simulink model "VU_NXTWay_Simple"  (Simulink 7.5)
settings: Solver=FixedStepDiscrete  SolverMode=SingleTasking  StartTime=0.0  StopTime=inf  FixedStep=0.004  RelTol=1e-3
PreLoadFcn:
  | param_plant, param_controller
values from neighbouring files (symbols this model uses):
  a_b = 0.8    [param_controller.m]
  a_d = 0.8    [param_controller.m]
  a_gc = 0.8    [param_controller.m]
  a_gd = 0.999    [param_controller.m]
  a_r = 0.996    [param_controller.m]
  gp_max = 100    [param_controller.m]
  k_f = KK(1, 1:4)    [param_controller.m]
  k_i = KK(1, 5)    [param_controller.m]
  k_phidot = 25    [param_controller.m]
  k_sync = 0.35    [param_controller.m]
  k_thetadot = 0.3 / R    [param_controller.m]
  pwm_gain = 1    [param_controller.m]
  sound_freq = 440    [param_controller.m]
  time_start = 1000    [param_controller.m]
  ts1 = 0.004    [param_controller.m]
libraries: lego_nxt_lib x8, simulink x3
settings Model: Creator=jpeytonj  LastModifiedBy=jpeytonj
settings DebuggingCC: SingleTaskRateTransMsg=warning  Int32ToFloatConvMsg=none  ParameterPrecisionLossMsg=none
settings RTWCC: SystemTargetFile=lrt.tlc  GenCodeOnly=on  TemplateMakefile=lrt_ecrobot.tmf  Description=Lego NXT Real-Time Target  ProcessScript=lrt_make_rtw_hook
settings STFCustomTargetCC: ModelReferenceCompliant=off  GeneratePreprocessorConditionals=Disable all  MatFileLogging=on  SystemTargetFile=lrt.tlc
settings GRTTargetCC: ModelReferenceCompliant=off  ParMdlRefBuildCompliant=off  CompOptLevelCompliant=off  ExtModeMexFile=ext_serial_win32_comm
settings CustomProperty: DataType=RTWOptions_EnumType_C__LegoMindstorms_VU-LRT_lrt_1codeGenType  Value=Integer-only
settings EnumStrPairs: String=Integer-only

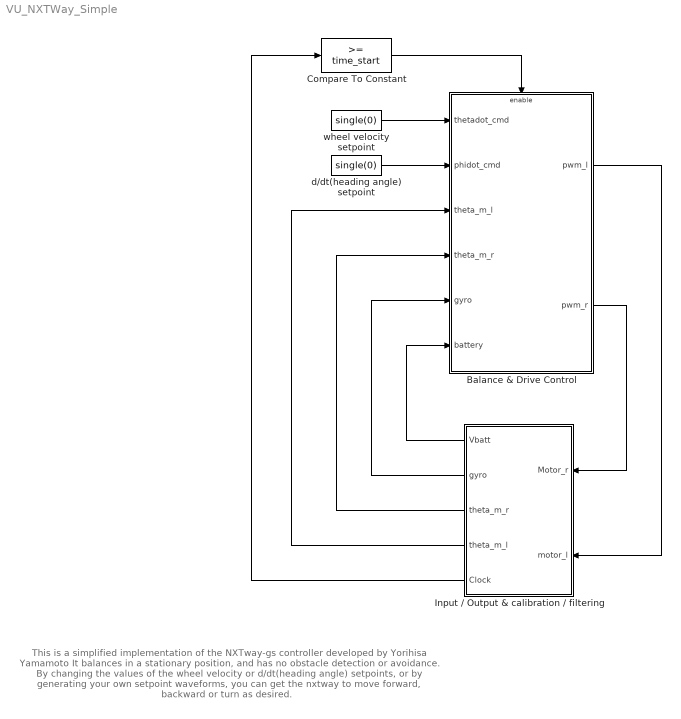
== system VU_NXTWay_Simple ==
  note: This is a simplified implementation of the NXTway-gs controller developed by Yorihisa Yamamoto
      | It balances in a stationary position, and has no obstacle detection or avoidance.
      |
      | By changing the values of the wheel velocity or d/dt(heading angle) setpoints, or by generating
      | your own setpoint waveforms, you can get the nxtway to move forward, backward or turn as desired.
  Balance & Drive Control : Subsystem
  Compare To Constant : simulink/Logic and Bit Operations/Compare To Constant  SystemSampleTime=-1  relop=>=  const=time_start  LogicOutDataTypeMode=boolean
  Input / Output & calibration / filtering : Subsystem
  d/dt(heading angle) setpoint : Constant  Value=single(0)  OutDataType=fixdt(1, 16)  OutScaling=2^0  SampleTime=ts1
  wheel velocity setpoint : Constant  Value=single(0)  OutDataType=fixdt(1, 16)  OutScaling=2^0  SampleTime=ts1
  wires:
  Input / Output & calibration / filtering/1(Vbatt) -> Balance & Drive Control/6(battery)
  Balance & Drive Control/2(pwm_r) -> Input / Output & calibration / filtering/1(Motor_r)
  Balance & Drive Control/1(pwm_l) -> Input / Output & calibration / filtering/2(motor_l)
  Compare To Constant/1 -> Balance & Drive Control/Enable
  Input / Output & calibration / filtering/5(Clock) -> Compare To Constant/1
  Input / Output & calibration / filtering/2(gyro) -> Balance & Drive Control/5(gyro)
  Input / Output & calibration / filtering/3(theta_m_r) -> Balance & Drive Control/4(theta_m_r)
  Input / Output & calibration / filtering/4(theta_m_l) -> Balance & Drive Control/3(theta_m_l)
  d/dt(heading angle) setpoint/1 -> Balance & Drive Control/2(phidot_cmd)
  wheel velocity setpoint/1 -> Balance & Drive Control/1(thetadot_cmd)

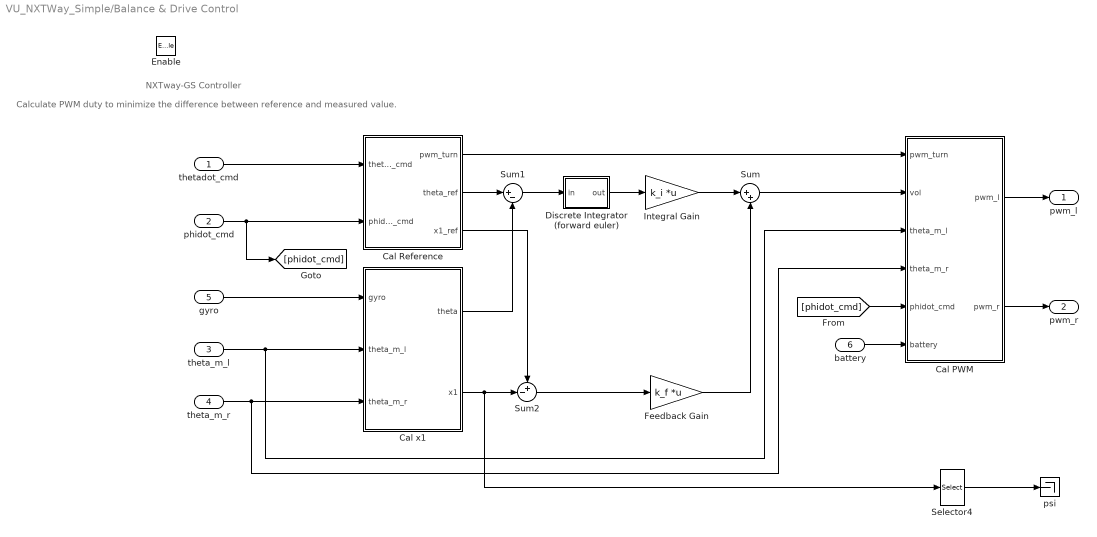
== system VU_NXTWay_Simple/Balance & Drive Control ==
  note: Calculate PWM duty to minimize the difference between reference and measured value.
  note: NXTway-GS Controller
  thetadot_cmd : Inport
  phidot_cmd : Inport  Port=2
  theta_m_l : Inport  Port=3
  theta_m_r : Inport  Port=4
  gyro : Inport  Port=5
  battery : Inport  Port=6
  Enable : EnablePort
  Cal PWM : Subsystem
  Cal Reference : Subsystem
  Cal x1 : Subsystem
  Discrete Integrator (forward euler) : Subsystem
  Feedback Gain : Gain  Gain=k_f  Multiplication=Matrix(K*u)  ParameterDataType=sfix(16)  ParameterScaling=2^0  OutDataType=sfix(16)  OutScaling=2^0  OutDataTypeStr=Inherit: Same as input  ParamDataTypeStr=Inherit: Same as input
  Integral Gain : Gain  Gain=k_i  Multiplication=Matrix(K*u)  ParameterDataType=sfix(16)  ParameterScaling=2^0  OutDataType=sfix(16)  OutScaling=2^0  OutDataTypeStr=Inherit: Same as input  ParamDataTypeStr=Inherit: Same as input
  Selector4 : Selector  InputPortWidth=4  IndexOptions=Index vector (dialog)  Indices=2  OutputSizes=1
  Sum : Sum  Inputs=|++  OutDataType=sfix(16)  OutScaling=2^0  OutDataTypeStr=Inherit: Same as first input
  Sum1 : Sum  Inputs=|+-  OutDataType=sfix(16)  OutScaling=2^0  OutDataTypeStr=Inherit: Same as first input
  Sum2 : Sum  Inputs=+-|  OutDataType=sfix(16)  OutScaling=2^0  OutDataTypeStr=Inherit: Same as first input
  psi : Terminator
  pwm_l : Outport
  pwm_r : Outport  Port=2
  wires:
  [phidot_cmd] -> Cal PWM/5(phidot_cmd)
  Selector4/1 -> psi/1
  Cal Reference/3(x1_ref) -> Sum2/1
  Sum2/1 -> Feedback Gain/1
  Cal x1/2(x1) -> Selector4/1, Sum2/2
  Integral Gain/1 -> Sum/1
  Discrete Integrator (forward euler)/1(out) -> Integral Gain/1
  Sum1/1 -> Discrete Integrator (forward euler)/1(in)
  Cal x1/1(theta) -> Sum1/2
  Cal Reference/2(theta_ref) -> Sum1/1
  Feedback Gain/1 -> Sum/2
  theta_m_r/1 -> Cal PWM/4(theta_m_r), Cal x1/3(theta_m_r)
  battery/1 -> Cal PWM/6(battery)
  Sum/1 -> Cal PWM/2(vol)
  phidot_cmd/1 -> [phidot_cmd], Cal Reference/2(phidot_cmd)
  thetadot_cmd/1 -> Cal Reference/1(thetadot_cmd)
  Cal Reference/1(pwm_turn) -> Cal PWM/1(pwm_turn)
  Cal PWM/1(pwm_l) -> pwm_l/1
  Cal PWM/2(pwm_r) -> pwm_r/1
  theta_m_l/1 -> Cal PWM/3(theta_m_l), Cal x1/2(theta_m_l)
  gyro/1 -> Cal x1/1(gyro)

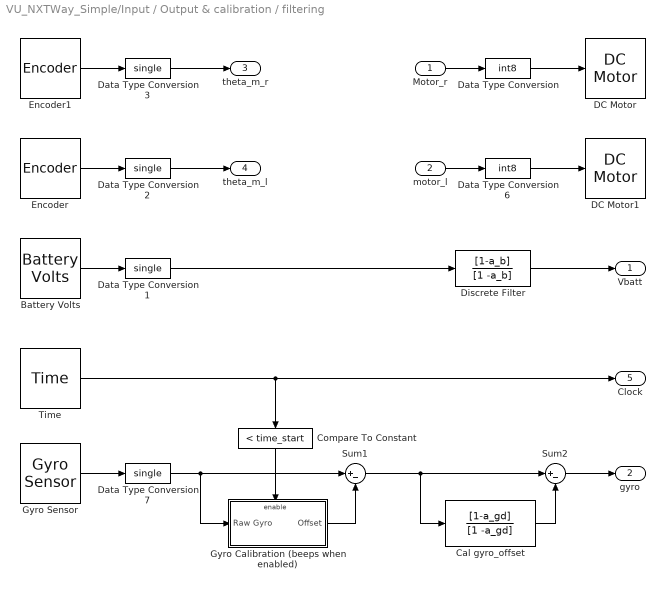
== system VU_NXTWay_Simple/Input / Output & calibration / filtering ==
  Motor_r : Inport
  motor_l : Inport  Port=2
  Battery Volts : lego_nxt_lib/Battery Volts  st=ts3
  Cal gyro_offset : DiscreteFilter  Numerator=[1-a_gd]  Denominator=[1 -a_gd]
  Compare To Constant : simulink/Logic and Bit Operations/Compare To Constant  SystemSampleTime=-1  relop=<  const=time_start  LogicOutDataTypeMode=boolean
  DC Motor : lego_nxt_lib/DC Motor  port=Port C  brake=Brake
  DC Motor1 : lego_nxt_lib/DC Motor  port=Port B  brake=Brake
  Data Type Conversion : DataTypeConversion  OutDataTypeMode=int8  OutDataType=sfix(16)  OutScaling=2^0  OutDataTypeStr=int8  RndMeth=Simplest
      settings: AttributesFormatString=Round = %<RndMeth>
  Data Type Conversion{1..3,7} (4 alike) : DataTypeConversion  OutDataTypeMode=single  OutDataType=sfix(16)  OutScaling=2^0  OutDataTypeStr=single  RndMeth=Simplest
      settings: AttributesFormatString=Round = %<RndMeth>
  Data Type Conversion6 : DataTypeConversion  OutDataTypeMode=int8  OutDataType=sfix(16)  OutScaling=2^0  OutDataTypeStr=int8  RndMeth=Simplest
      settings: AttributesFormatString=Round = %<RndMeth>
  Discrete Filter : DiscreteFilter  Numerator=[1-a_b]  Denominator=[1 -a_b]
  Encoder : lego_nxt_lib/Encoder  port=Port B  st=ts1
  Encoder1 : lego_nxt_lib/Encoder  port=Port C  st=ts1
  Gyro Calibration (beeps when enabled) : Subsystem  TreatAsAtomicUnit=on
  Gyro Sensor : lego_nxt_lib/Gyro Sensor  port=Port 3  st=ts1
  Sum1 : Sum  Inputs=|+-  OutDataType=sfix(16)  OutScaling=2^0  OutDataTypeStr=Inherit: Same as first input
  Sum2 : Sum  Inputs=|+-  OutDataType=sfix(16)  OutScaling=2^0  OutDataTypeStr=Inherit: Same as first input
  Time : lego_nxt_lib/Time  st=ts1
  Vbatt : Outport
  gyro : Outport  Port=2
  theta_m_r : Outport  Port=3
  theta_m_l : Outport  Port=4
  Clock : Outport  Port=5
  wires:
  Gyro Sensor/1 -> Data Type Conversion7/1
  Encoder/1 -> Data Type Conversion2/1
  Encoder1/1 -> Data Type Conversion3/1
  Battery Volts/1 -> Data Type Conversion1/1
  motor_l/1 -> Data Type Conversion6/1
  Motor_r/1 -> Data Type Conversion/1
  Time/1 -> Clock/1, Compare To Constant/1
  Discrete Filter/1 -> Vbatt/1
  Data Type Conversion1/1 -> Discrete Filter/1
  Sum2/1 -> gyro/1
  Data Type Conversion7/1 -> Gyro Calibration (beeps when enabled)/1(Raw Gyro), Sum1/1
  Sum1/1 -> Cal gyro_offset/1, Sum2/1
  Compare To Constant/1 -> Gyro Calibration (beeps when enabled)/Enable
  Cal gyro_offset/1 -> Sum2/2
  Gyro Calibration (beeps when enabled)/1(Offset) -> Sum1/2
  Data Type Conversion2/1 -> theta_m_l/1
  Data Type Conversion3/1 -> theta_m_r/1
  Data Type Conversion/1 -> DC Motor/1
  Data Type Conversion6/1 -> DC Motor1/1

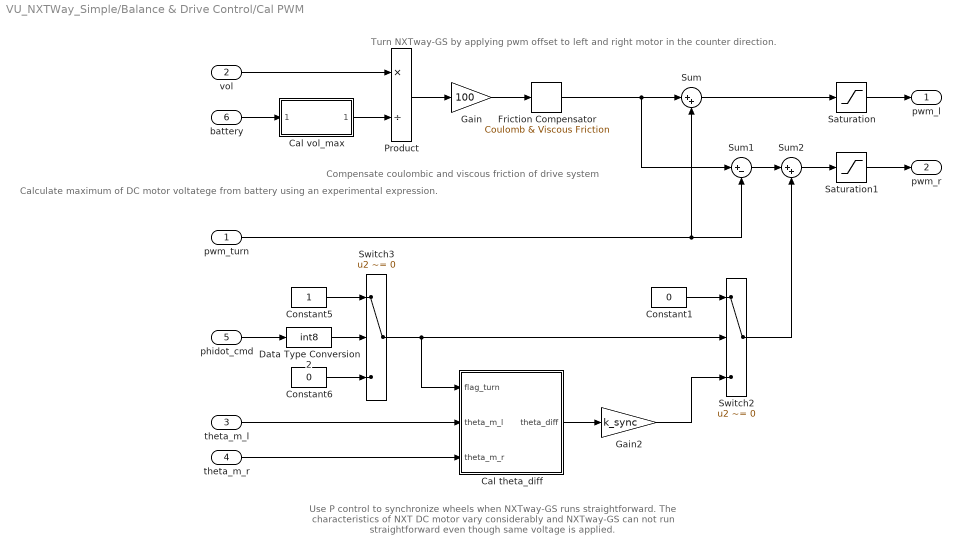
== system VU_NXTWay_Simple/Balance & Drive Control/Cal PWM ==
  note: Compensate coulombic and
      | viscous friction of drive system
  note: Turn NXTway-GS by applying pwm offset
      | to left and right motor in the counter direction.
  note: Use P control to synchronize wheels when NXTway-GS runs straightforward.
      | The characteristics of NXT DC motor vary considerably and NXTway-GS can not
      | run straightforward even though same voltage is applied.
  note: Calculate maximum of DC motor
      | voltatege from battery using an
      | experimental expression.
  pwm_turn : Inport
  vol : Inport  Port=2  OutDataType=sfix(16)  OutScaling=2^0
  theta_m_l : Inport  Port=3  OutDataType=sfix(16)  OutScaling=2^0
  theta_m_r : Inport  Port=4  OutDataType=sfix(16)  OutScaling=2^0
  phidot_cmd : Inport  Port=5
  battery : Inport  Port=6  OutDataType=sfix(16)  OutScaling=2^0
  Cal theta_diff : Subsystem
  Cal vol_max : Subsystem
  Constant1 : Constant  Value=0  OutDataTypeMode=single  OutDataType=sfix(16)  OutScaling=2^0  OutDataTypeStr=single  SampleTime=ts1
      settings: AttributesFormatString=DataType = %<OutDataTypeStr>
  Constant5 : Constant  OutDataTypeMode=boolean  OutDataType=sfix(16)  OutScaling=2^0  OutDataTypeStr=boolean  SampleTime=ts1
      settings: AttributesFormatString=DataType = %<OutDataTypeStr>
  Constant6 : Constant  Value=0  OutDataTypeMode=boolean  OutDataType=sfix(16)  OutScaling=2^0  OutDataTypeStr=boolean  SampleTime=ts1
      settings: AttributesFormatString=DataType = %<OutDataTypeStr>
  Data Type Conversion2 : DataTypeConversion  OutDataTypeMode=int8  OutDataType=sfix(16)  OutScaling=2^0  OutDataTypeStr=int8  RndMeth=Simplest
      settings: AttributesFormatString=Round = %<RndMeth>
  Friction Compensator : simulink/Discontinuities/Coulomb & Viscous Friction  SystemSampleTime=-1  offset=pwm_offset  gain=pwm_gain
      settings: AttributesFormatString=gain = %<gain>\noffset = %<offset>
  Gain : Gain  Gain=100  ParameterDataType=sfix(16)  ParameterScaling=2^0  OutDataType=sfix(16)  OutScaling=2^0  OutDataTypeStr=Inherit: Same as input  ParamDataTypeStr=Inherit: Same as input
  Gain2 : Gain  Gain=k_sync  ParameterDataType=sfix(16)  ParameterScaling=2^0  OutDataType=sfix(16)  OutScaling=2^0  OutDataTypeStr=Inherit: Same as input  ParamDataTypeStr=Inherit: Same as input
  Product : Product  Inputs=*/  OutDataType=sfix(16)  OutScaling=2^0  RndMeth=Simplest  OutDataTypeStr=Inherit: Same as first input
  Saturation : Saturate  UpperLimit=100  LowerLimit=-100
      settings: AttributesFormatString=max = %<UpperLimit>\nmin = %<LowerLimit>
  Saturation1 : Saturate  UpperLimit=100  LowerLimit=-100
      settings: AttributesFormatString=max = %<UpperLimit>\nmin = %<LowerLimit>
  Sum : Sum  Inputs=|++  OutDataType=sfix(16)  OutScaling=2^0  OutDataTypeStr=Inherit: Same as first input
  Sum1 : Sum  Inputs=|+-  OutDataType=sfix(16)  OutScaling=2^0  OutDataTypeStr=Inherit: Same as first input
  Sum2 : Sum  Inputs=|++  OutDataType=sfix(16)  OutScaling=2^0  OutDataTypeStr=Inherit: Same as first input
  Switch2 : Switch  Criteria=u2 ~= 0  OutDataType=sfix(16)  OutScaling=2^0
  Switch3 : Switch  Criteria=u2 ~= 0  OutDataType=sfix(16)  OutScaling=2^0
  pwm_l : Outport  OutDataType=sfix(16)  OutScaling=2^0
  pwm_r : Outport  Port=2  OutDataType=sfix(16)  OutScaling=2^0
  wires:
  Data Type Conversion2/1 -> Switch3/2
  phidot_cmd/1 -> Data Type Conversion2/1
  Constant6/1 -> Switch3/3
  Constant5/1 -> Switch3/1
  theta_m_r/1 -> Cal theta_diff/3(theta_m_r)
  theta_m_l/1 -> Cal theta_diff/2(theta_m_l)
  Friction Compensator/1 -> Sum/1, Sum1/1
  Sum2/1 -> Saturation1/1
  Sum1/1 -> Sum2/1
  Cal vol_max/1(vol_max) -> Product/2
  battery/1 -> Cal vol_max/1(battery)
  Gain2/1 -> Switch2/3
  Constant1/1 -> Switch2/1
  Switch3/1 -> Cal theta_diff/1(flag_turn), Switch2/2
  Cal theta_diff/1(theta_diff) -> Gain2/1
  Product/1 -> Gain/1
  vol/1 -> Product/1
  Saturation/1 -> pwm_l/1
  Saturation1/1 -> pwm_r/1
  Gain/1 -> Friction Compensator/1
  pwm_turn/1 -> Sum1/2, Sum/2
  Sum/1 -> Saturation/1
  Switch2/1 -> Sum2/2

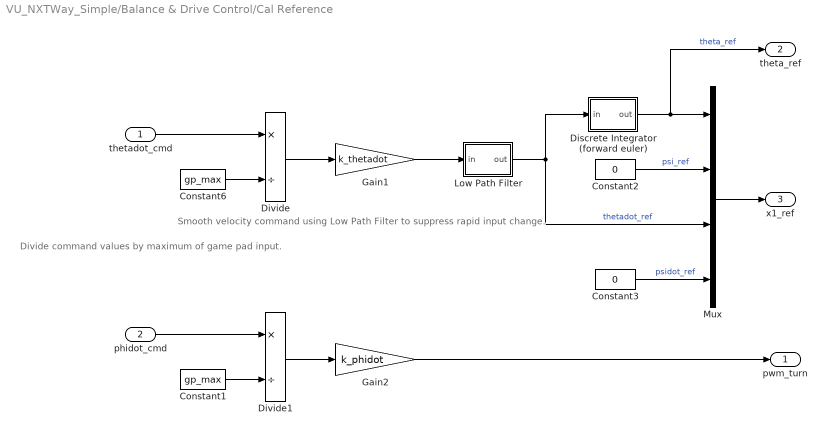
== system VU_NXTWay_Simple/Balance & Drive Control/Cal Reference ==
  note: Smooth velocity command
      | using Low Path Filter to
      | suppress rapid input change.
  note: Divide command values by
      | maximum of game pad input.
  thetadot_cmd : Inport
  phidot_cmd : Inport  Port=2
  Constant1 : Constant  Value=gp_max  VectorParams1D=off  OutDataTypeMode=int8  OutDataType=FIXDT  OutScaling=2^0  OutDataTypeStr=int8  SampleTime=ts1
      settings: AttributesFormatString=DataType = %<OutDataTypeStr>
  Constant2 : Constant  Value=0  VectorParams1D=off  OutDataTypeMode=single  OutDataType=FIXDT  OutScaling=2^0  OutDataTypeStr=single  SampleTime=ts1
      settings: AttributesFormatString=DataType = %<OutDataTypeStr>
  Constant3 : Constant  Value=0  VectorParams1D=off  OutDataTypeMode=single  OutDataType=FIXDT  OutScaling=2^0  OutDataTypeStr=single  SampleTime=ts1
      settings: AttributesFormatString=DataType = %<OutDataTypeStr>
  Constant6 : Constant  Value=gp_max  VectorParams1D=off  OutDataTypeMode=int8  OutDataType=FIXDT  OutScaling=2^0  OutDataTypeStr=int8  SampleTime=ts1
      settings: AttributesFormatString=DataType = %<OutDataTypeStr>
  Discrete Integrator (forward euler) : Subsystem
  Divide : Product  Inputs=*/  OutDataType=sfix(16)  OutScaling=2^-10  RndMeth=Simplest  OutDataTypeStr=Inherit: Same as first input
  Divide1 : Product  Inputs=*/  OutDataType=sfix(16)  OutScaling=2^-10  RndMeth=Simplest  OutDataTypeStr=Inherit: Same as first input
  Gain1 : Gain  Gain=k_thetadot  ParameterDataType=sfix(16)  ParameterScaling=2^0  OutDataType=sfix(16)  OutScaling=2^0  OutDataTypeStr=Inherit: Same as input  ParamDataTypeStr=Inherit: Same as input
  Gain2 : Gain  Gain=k_phidot  ParameterDataType=sfix(16)  ParameterScaling=2^0  OutDataType=sfix(16)  OutScaling=2^0  OutDataTypeStr=Inherit: Same as input  ParamDataTypeStr=Inherit: Same as input
  Low Path Filter : Subsystem
  Mux : Mux
  pwm_turn : Outport
  theta_ref : Outport  Port=2
  x1_ref : Outport  Port=3
  wires:
  Constant6/1 -> Divide/2
  Low Path Filter/1(out) -> Mux/3, Discrete Integrator (forward euler)/1(in)  "thetadot_ref"
  Constant3/1 -> Mux/4  "psidot_ref"
  Constant2/1 -> Mux/2  "psi_ref"
  Discrete Integrator (forward euler)/1(out) -> Mux/1, theta_ref/1  "theta_ref"
  Mux/1 -> x1_ref/1
  Divide1/1 -> Gain2/1
  Constant1/1 -> Divide1/2
  Gain2/1 -> pwm_turn/1
  Divide/1 -> Gain1/1
  thetadot_cmd/1 -> Divide/1
  Gain1/1 -> Low Path Filter/1(in)
  phidot_cmd/1 -> Divide1/1

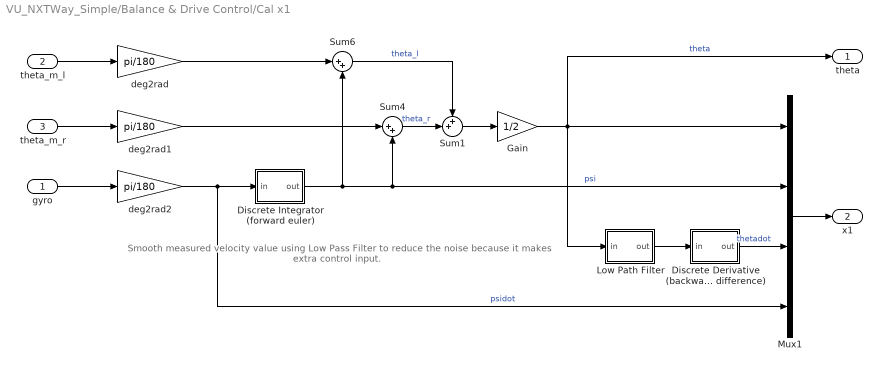
== system VU_NXTWay_Simple/Balance & Drive Control/Cal x1 ==
  note: Smooth measured velocity value using
      | Low Pass Filter to reduce the noise
      | because it makes extra control input.
  gyro : Inport  OutDataType=sfix(16)  OutScaling=2^0
  theta_m_l : Inport  Port=2  OutDataType=sfix(16)  OutScaling=2^0
  theta_m_r : Inport  Port=3  OutDataType=sfix(16)  OutScaling=2^0
  Discrete Derivative (backward difference) : Subsystem
  Discrete Integrator (forward euler) : Subsystem
  Gain : Gain  Gain=1/2  ParameterDataType=sfix(16)  ParameterScaling=2^0  OutDataType=sfix(16)  OutScaling=2^0  OutDataTypeStr=Inherit: Same as input  ParamDataTypeStr=Inherit: Same as input
  Low Path Filter : Subsystem
  Mux1 : Mux
  Sum1 : Sum  Inputs=++|  OutDataType=sfix(16)  OutScaling=2^0  OutDataTypeStr=Inherit: Same as first input
  Sum4 : Sum  Inputs=|++  OutDataType=sfix(16)  OutScaling=2^0  OutDataTypeStr=Inherit: Same as first input
  Sum6 : Sum  Inputs=|++  OutDataType=sfix(16)  OutScaling=2^0  OutDataTypeStr=Inherit: Same as first input
  deg2rad : Gain  Gain=pi/180  ParameterDataType=sfix(16)  ParameterScaling=2^0  OutDataType=sfix(16)  OutScaling=2^0  OutDataTypeStr=Inherit: Same as input  ParamDataTypeStr=Inherit: Same as input
  deg2rad1 : Gain  Gain=pi/180  ParameterDataType=sfix(16)  ParameterScaling=2^0  OutDataType=sfix(16)  OutScaling=2^0  OutDataTypeStr=Inherit: Same as input  ParamDataTypeStr=Inherit: Same as input
  deg2rad2 : Gain  Gain=pi/180  ParameterDataType=sfix(16)  ParameterScaling=2^0  OutDataType=sfix(16)  OutScaling=2^0  OutDataTypeStr=Inherit: Same as input  ParamDataTypeStr=Inherit: Same as input
  theta : Outport  OutDataType=sfix(16)  OutScaling=2^0
  x1 : Outport  Port=2  OutDataType=sfix(16)  OutScaling=2^0
  wires:
  Gain/1 -> Low Path Filter/1(in), Mux1/1, theta/1  "theta"
  Low Path Filter/1(out) -> Discrete Derivative (backward difference)/1(in)
  deg2rad2/1 -> Mux1/4, Discrete Integrator (forward euler)/1(in)  "psidot"
  Sum1/1 -> Gain/1
  Sum4/1 -> Sum1/2  "theta_r"
  Sum6/1 -> Sum1/1  "theta_l"
  Discrete Derivative (backward difference)/1(out) -> Mux1/3  "thetadot"
  theta_m_r/1 -> deg2rad1/1
  theta_m_l/1 -> deg2rad/1
  deg2rad/1 -> Sum6/1
  Discrete Integrator (forward euler)/1(out) -> Mux1/2, Sum4/2, Sum6/2  "psi"
  Mux1/1 -> x1/1
  deg2rad1/1 -> Sum4/1
  gyro/1 -> deg2rad2/1

== system VU_NXTWay_Simple/Balance & Drive Control/Discrete Integrator (forward euler) ==
  in : Inport  OutDataType=sfix(16)  OutScaling=2^0
  Gain : Gain  Gain=ts1  ParameterDataType=sfix(16)  ParameterScaling=2^0  OutDataType=sfix(16)  OutScaling=2^0  OutDataTypeStr=Inherit: Same as input  ParamDataTypeStr=Inherit: Same as input
  Sum : Sum  Inputs=|++  OutDataType=sfix(16)  OutScaling=2^0  OutDataTypeStr=Inherit: Same as first input
  Unit Delay : UnitDelay  SampleTime=-1
  out : Outport  OutDataType=sfix(16)  OutScaling=2^0
  wires:
  in/1 -> Gain/1
  Sum/1 -> Unit Delay/1
  Gain/1 -> Sum/1
  Unit Delay/1 -> out/1, Sum/2

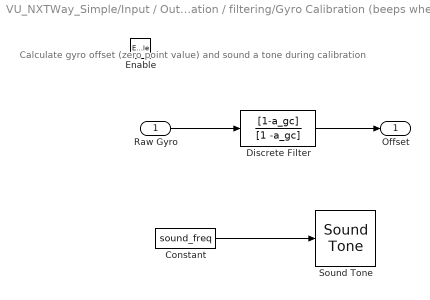
== system VU_NXTWay_Simple/Input / Output & calibration / filtering/Gyro Calibration (beeps when enabled) ==
  note: Calculate gyro offset (zero point value)
      | and sound a tone during calibration
  Raw Gyro : Inport  OutDataType=fixdt(1, 16)  OutScaling=2^0
  Enable : EnablePort
  Constant : Constant  Value=sound_freq  OutDataTypeMode=uint32  OutDataType=sfix(16)  OutScaling=2^0  OutDataTypeStr=uint32  SampleTime=0.2
      settings: AttributesFormatString=DataType = %<OutDataTypeStr>
  Discrete Filter : DiscreteFilter  Numerator=[1-a_gc]  Denominator=[1 -a_gc]
  Sound Tone : lego_nxt_lib/Sound Tone  SystemSampleTime=-1  freqsrc=External  freq=0  volsrc=Internal  vol=20
  Offset : Outport  OutDataType=fixdt(1, 16)  OutScaling=2^0
  wires:
  Discrete Filter/1 -> Offset/1
  Raw Gyro/1 -> Discrete Filter/1
  Constant/1 -> Sound Tone/1

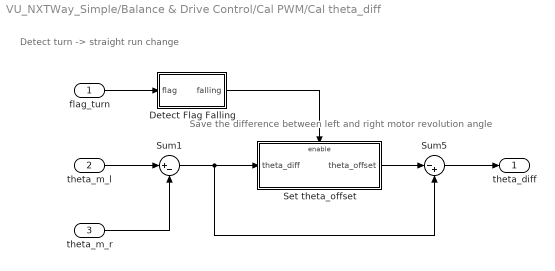
== system VU_NXTWay_Simple/Balance & Drive Control/Cal PWM/Cal theta_diff ==
  note: Save the difference between
      | left and right motor revolution angle
  note: Detect turn -> straight run change
  flag_turn : Inport
  theta_m_l : Inport  Port=2
  theta_m_r : Inport  Port=3
  Detect Flag Falling : Subsystem
  Set theta_offset : Subsystem
  Sum1 : Sum  Inputs=|+-  OutDataType=sfix(16)  OutScaling=2^0  OutDataTypeStr=Inherit: Same as first input
  Sum5 : Sum  Inputs=|-+  OutDataType=sfix(16)  OutScaling=2^0  OutDataTypeStr=Inherit: Same as first input
  theta_diff : Outport
  wires:
  Set theta_offset/1(theta_offset) -> Sum5/1
  theta_m_r/1 -> Sum1/2
  theta_m_l/1 -> Sum1/1
  Sum1/1 -> Sum5/2, Set theta_offset/1(theta_diff)
  Detect Flag Falling/1(falling) -> Set theta_offset/Enable
  Sum5/1 -> theta_diff/1
  flag_turn/1 -> Detect Flag Falling/1(flag)

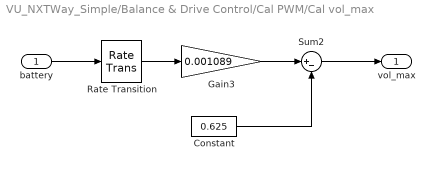
== system VU_NXTWay_Simple/Balance & Drive Control/Cal PWM/Cal vol_max ==
  battery : Inport
  Constant : Constant  Value=0.625  OutDataTypeMode=single  OutDataType=sfix(16)  OutScaling=2^0  OutDataTypeStr=single  SampleTime=ts1
      settings: AttributesFormatString=DataType = %<OutDataTypeStr>
  Gain3 : Gain  Gain=0.001089  ParameterDataType=sfix(16)  ParameterScaling=2^0  OutDataType=sfix(16)  OutScaling=2^0  SampleTime=ts1  OutDataTypeStr=Inherit: Same as input  ParamDataTypeStr=Inherit: Same as input
  Rate Transition : RateTransition  OutPortSampleTimeOpt=Inherit
  Sum2 : Sum  Inputs=|+-  OutDataType=sfix(16)  OutScaling=2^0  OutDataTypeStr=Inherit: Same as first input
  vol_max : Outport
  wires:
  Gain3/1 -> Sum2/1
  Sum2/1 -> vol_max/1
  Constant/1 -> Sum2/2
  battery/1 -> Rate Transition/1
  Rate Transition/1 -> Gain3/1

== system VU_NXTWay_Simple/Balance & Drive Control/Cal Reference/Discrete Integrator (forward euler) ==
  in : Inport  OutDataType=sfix(16)  OutScaling=2^0
  Gain : Gain  Gain=ts1  ParameterDataType=sfix(16)  ParameterScaling=2^0  OutDataType=sfix(16)  OutScaling=2^0  OutDataTypeStr=Inherit: Same as input  ParamDataTypeStr=Inherit: Same as input
  Sum : Sum  Inputs=|++  OutDataType=sfix(16)  OutScaling=2^0  OutDataTypeStr=Inherit: Same as first input
  Unit Delay : UnitDelay  SampleTime=-1
  out : Outport  OutDataType=sfix(16)  OutScaling=2^0
  wires:
  in/1 -> Gain/1
  Sum/1 -> Unit Delay/1
  Gain/1 -> Sum/1
  Unit Delay/1 -> out/1, Sum/2

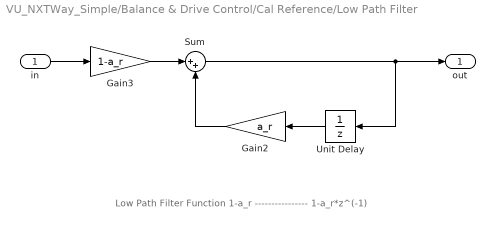
== system VU_NXTWay_Simple/Balance & Drive Control/Cal Reference/Low Path Filter ==
  note: Low Path Filter Function
      |               1-a_r
      |          ----------------
      |          1-a_r*z^(-1)
  in : Inport
  Gain2 : Gain  Gain=a_r  ParameterDataType=sfix(16)  ParameterScaling=2^0  OutDataType=sfix(16)  OutScaling=2^0  OutDataTypeStr=Inherit: Same as input  ParamDataTypeStr=Inherit: Same as input
  Gain3 : Gain  Gain=1-a_r  ParameterDataType=sfix(16)  ParameterScaling=2^0  OutDataType=sfix(16)  OutScaling=2^0  OutDataTypeStr=Inherit: Same as input  ParamDataTypeStr=Inherit: Same as input
  Sum : Sum  Inputs=|++  OutDataType=sfix(16)  OutScaling=2^0  OutDataTypeStr=Inherit: Same as first input
  Unit Delay : UnitDelay  SampleTime=-1
  out : Outport
  wires:
  in/1 -> Gain3/1
  Gain3/1 -> Sum/1
  Gain2/1 -> Sum/2
  Unit Delay/1 -> Gain2/1
  Sum/1 -> out/1, Unit Delay/1

== system VU_NXTWay_Simple/Balance & Drive Control/Cal x1/Discrete Derivative (backward difference) ==
  in : Inport  OutDataType=sfix(16)  OutScaling=2^0
  Gain : Gain  Gain=1/ts1  ParameterDataType=sfix(16)  ParameterScaling=2^0  OutDataType=sfix(16)  OutScaling=2^0  OutDataTypeStr=Inherit: Same as input  ParamDataTypeStr=Inherit: Same as input
  Sum : Sum  Inputs=|+-  OutDataType=sfix(16)  OutScaling=2^0  OutDataTypeStr=Inherit: Same as first input
  Unit Delay : UnitDelay  SampleTime=-1
  out : Outport  OutDataType=sfix(16)  OutScaling=2^0
  wires:
  Gain/1 -> out/1
  in/1 -> Sum/1, Unit Delay/1
  Unit Delay/1 -> Sum/2
  Sum/1 -> Gain/1

== system VU_NXTWay_Simple/Balance & Drive Control/Cal x1/Discrete Integrator (forward euler) ==
  in : Inport  OutDataType=sfix(16)  OutScaling=2^0
  Gain : Gain  Gain=ts1  ParameterDataType=sfix(16)  ParameterScaling=2^0  OutDataType=sfix(16)  OutScaling=2^0  OutDataTypeStr=Inherit: Same as input  ParamDataTypeStr=Inherit: Same as input
  Sum : Sum  Inputs=|++  OutDataType=sfix(16)  OutScaling=2^0  OutDataTypeStr=Inherit: Same as first input
  Unit Delay : UnitDelay  SampleTime=-1
  out : Outport  OutDataType=sfix(16)  OutScaling=2^0
  wires:
  Unit Delay/1 -> Sum/2, out/1
  Gain/1 -> Sum/1
  Sum/1 -> Unit Delay/1
  in/1 -> Gain/1

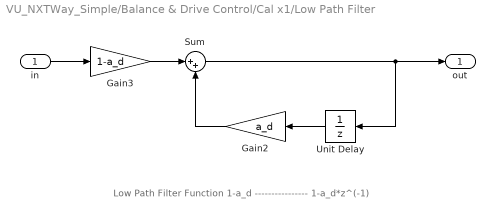
== system VU_NXTWay_Simple/Balance & Drive Control/Cal x1/Low Path Filter ==
  note: Low Path Filter Function
      |               1-a_d
      |          ----------------
      |          1-a_d*z^(-1)
  in : Inport
  Gain2 : Gain  Gain=a_d  ParameterDataType=sfix(16)  ParameterScaling=2^0  OutDataType=sfix(16)  OutScaling=2^0  OutDataTypeStr=Inherit: Same as input  ParamDataTypeStr=Inherit: Same as input
  Gain3 : Gain  Gain=1-a_d  ParameterDataType=sfix(16)  ParameterScaling=2^0  OutDataType=sfix(16)  OutScaling=2^0  OutDataTypeStr=Inherit: Same as input  ParamDataTypeStr=Inherit: Same as input
  Sum : Sum  Inputs=|++  OutDataType=sfix(16)  OutScaling=2^0  OutDataTypeStr=Inherit: Same as first input
  Unit Delay : UnitDelay  SampleTime=-1
  out : Outport
  wires:
  in/1 -> Gain3/1
  Gain3/1 -> Sum/1
  Gain2/1 -> Sum/2
  Unit Delay/1 -> Gain2/1
  Sum/1 -> out/1, Unit Delay/1

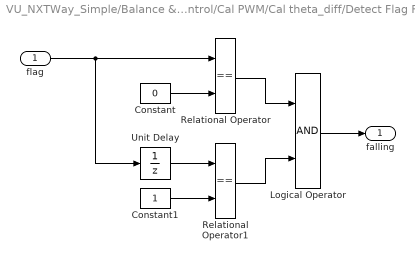
== system VU_NXTWay_Simple/Balance & Drive Control/Cal PWM/Cal theta_diff/Detect Flag Falling ==
  flag : Inport  OutDataType=sfix(16)  OutScaling=2^0
  Constant : Constant  Value=0  VectorParams1D=off  OutDataTypeMode=boolean  OutDataType=FIXDT  OutScaling=2^0  OutDataTypeStr=boolean  SampleTime=ts1
      settings: AttributesFormatString=DataType = %<OutDataTypeStr>
  Constant1 : Constant  VectorParams1D=off  OutDataTypeMode=boolean  OutDataType=FIXDT  OutScaling=2^0  OutDataTypeStr=boolean  SampleTime=ts1
      settings: AttributesFormatString=DataType = %<OutDataTypeStr>
  Logical Operator : Logic  AllPortsSameDT=off  OutDataTypeMode=boolean  OutDataTypeStr=boolean
  Relational Operator : RelationalOperator  Operator===  LogicOutDataTypeMode=boolean  OutDataTypeStr=boolean
  Relational Operator1 : RelationalOperator  Operator===  LogicOutDataTypeMode=boolean  OutDataTypeStr=boolean
  Unit Delay : UnitDelay  SampleTime=-1
  falling : Outport  OutDataType=sfix(16)  OutScaling=2^0
  wires:
  Logical Operator/1 -> falling/1
  Relational Operator1/1 -> Logical Operator/2
  Relational Operator/1 -> Logical Operator/1
  Constant1/1 -> Relational Operator1/2
  Unit Delay/1 -> Relational Operator1/1
  Constant/1 -> Relational Operator/2
  flag/1 -> Relational Operator/1, Unit Delay/1

== system VU_NXTWay_Simple/Balance & Drive Control/Cal PWM/Cal theta_diff/Set theta_offset ==
  theta_diff : Inport
  Enable : EnablePort
  theta_offset : Outport
  wires:
  theta_diff/1 -> theta_offset/1
